simulink model "day04p2"  (R2026a)
settings: Solver=VariableStepAuto  StopTime=inf
undefined symbols (not defined in the file): DiscIntNeverNeededParam
libraries: simulink x6
(part 2 of 2)

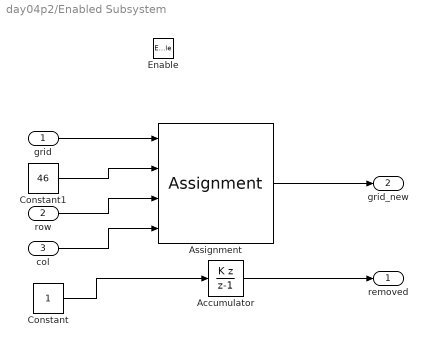
== system day04p2/Enabled Subsystem ==
  grid : Inport
  row : Inport  Port=2
  col : Inport  Port=3
  Enable : EnablePort
  Accumulator : DiscreteIntegrator  IntegratorMethod=Accumulation: Backward Euler  SampleTime=-1  ICPrevOutput=DiscIntNeverNeededParam  ICPrevScaledInput=DiscIntNeverNeededParam
  Assignment : Assignment  NumberOfDimensions=2  DiagnosticForDimensions=Warning  IndexOptions=Index vector (port),Index vector (port)  Indices=1,1  OutputSizes=1,1
  Constant : Constant
  Constant1 : Constant  Value=46
  removed : Outport
  grid_new : Outport  Port=2
  wires:
  Constant/1 -> Accumulator/1
  Accumulator/1 -> removed/1
  grid/1 -> Assignment/1
  Assignment/1 -> grid_new/1
  Constant1/1 -> Assignment/2
  row/1 -> Assignment/3
  col/1 -> Assignment/4

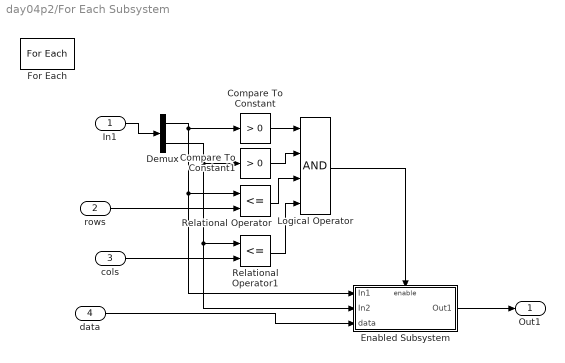
== system day04p2/For Each Subsystem ==
  In1 : Inport  Partition=on  PartitionDimension=1  PartitionWidth=1  PartitionOffset=0
  rows : Inport  Port=2
  cols : Inport  Port=3
  data : Inport  Port=4
  Compare To Constant : simulink/Logic and Bit Operations/Compare To Constant  relop=>  const=0  OutDataTypeStr=boolean
  Compare To Constant1 : simulink/Logic and Bit Operations/Compare To Constant  relop=>  const=0  OutDataTypeStr=boolean
  Demux : Demux  Outputs=2
  Enabled Subsystem : Subsystem  TreatAsAtomicUnit=on
  For Each : ForEach  DisableCoverage=on
  Logical Operator : Logic  Inputs=4  AllPortsSameDT=off  OutDataTypeStr=boolean
  Relational Operator : RelationalOperator  Operator=<=  OutDataTypeStr=boolean  RndMeth=Simplest  InputSameDT=off
  Relational Operator1 : RelationalOperator  Operator=<=  OutDataTypeStr=boolean  RndMeth=Simplest  InputSameDT=off
  Out1 : Outport  ConcatenationDimension=1
  wires:
  In1/1 -> Demux/1
  Demux/1 -> Enabled Subsystem/1(In1), Relational Operator/1, Compare To Constant/1
  Demux/2 -> Enabled Subsystem/2(In2), Relational Operator1/1, Compare To Constant1/1
  rows/1 -> Relational Operator/2
  cols/1 -> Relational Operator1/2
  Compare To Constant/1 -> Logical Operator/1
  Compare To Constant1/1 -> Logical Operator/2
  Relational Operator/1 -> Logical Operator/3
  Relational Operator1/1 -> Logical Operator/4
  data/1 -> Enabled Subsystem/3(data)
  Logical Operator/1 -> Enabled Subsystem/Enable
  Enabled Subsystem/1(Out1) -> Out1/1

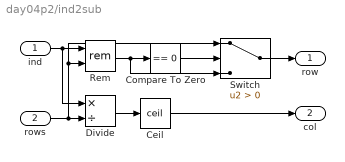
== system day04p2/ind2sub ==
  ind : Inport
  rows : Inport  Port=2
  Ceil : Rounding  Operator=ceil
  Compare To Zero : simulink/Logic and Bit Operations/Compare To Zero  relop===  OutDataTypeStr=boolean
  Divide : Product  Inputs=*/
  Rem : Math  Operator=rem
  Switch : Switch  Criteria=u2 > Threshold  SaturateOnIntegerOverflow=off  InputSameDT=off
  row : Outport
  col : Outport  Port=2
  wires:
  ind/1 -> Rem/1, Divide/1
  rows/1 -> Rem/2, Switch/1, Divide/2
  Divide/1 -> Ceil/1
  Ceil/1 -> col/1
  Rem/1 -> Switch/3, Compare To Zero/1
  Compare To Zero/1 -> Switch/2
  Switch/1 -> row/1

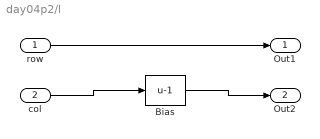
== system day04p2/l ==
  row : Inport
  col : Inport  Port=2
  Bias : Bias  Bias=-1  SaturateOnIntegerOverflow=off
  Out1 : Outport
  Out2 : Outport  Port=2
  wires:
  row/1 -> Out1/1
  col/1 -> Bias/1
  Bias/1 -> Out2/1

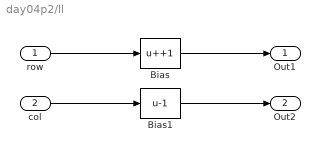
== system day04p2/ll ==
  row : Inport
  col : Inport  Port=2
  Bias : Bias  Bias=+1  SaturateOnIntegerOverflow=off
  Bias1 : Bias  Bias=-1  SaturateOnIntegerOverflow=off
  Out1 : Outport
  Out2 : Outport  Port=2
  wires:
  row/1 -> Bias/1
  Bias/1 -> Out1/1
  col/1 -> Bias1/1
  Bias1/1 -> Out2/1

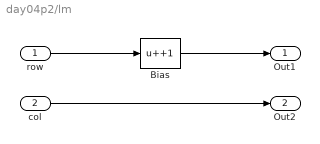
== system day04p2/lm ==
  row : Inport
  col : Inport  Port=2
  Bias : Bias  Bias=+1  SaturateOnIntegerOverflow=off
  Out1 : Outport
  Out2 : Outport  Port=2
  wires:
  row/1 -> Bias/1
  Bias/1 -> Out1/1
  col/1 -> Out2/1

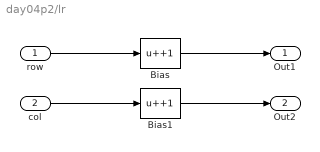
== system day04p2/lr ==
  row : Inport
  col : Inport  Port=2
  Bias : Bias  Bias=+1  SaturateOnIntegerOverflow=off
  Bias1 : Bias  Bias=+1  SaturateOnIntegerOverflow=off
  Out1 : Outport
  Out2 : Outport  Port=2
  wires:
  row/1 -> Bias/1
  Bias/1 -> Out1/1
  col/1 -> Bias1/1
  Bias1/1 -> Out2/1

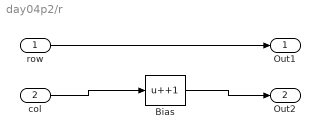
== system day04p2/r ==
  row : Inport
  col : Inport  Port=2
  Bias : Bias  Bias=+1  SaturateOnIntegerOverflow=off
  Out1 : Outport
  Out2 : Outport  Port=2
  wires:
  col/1 -> Bias/1
  Bias/1 -> Out2/1
  row/1 -> Out1/1

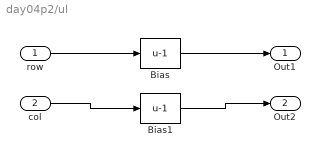
== system day04p2/ul ==
  row : Inport
  col : Inport  Port=2
  Bias : Bias  Bias=-1  SaturateOnIntegerOverflow=off
  Bias1 : Bias  Bias=-1  SaturateOnIntegerOverflow=off
  Out1 : Outport
  Out2 : Outport  Port=2
  wires:
  row/1 -> Bias/1
  Bias/1 -> Out1/1
  col/1 -> Bias1/1
  Bias1/1 -> Out2/1

== system day04p2/um ==
  row : Inport
  col : Inport  Port=2
  Bias : Bias  Bias=-1  SaturateOnIntegerOverflow=off
  Out1 : Outport
  Out2 : Outport  Port=2
  wires:
  col/1 -> Out2/1
  row/1 -> Bias/1
  Bias/1 -> Out1/1

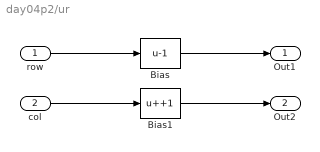
== system day04p2/ur ==
  row : Inport
  col : Inport  Port=2
  Bias : Bias  Bias=-1  SaturateOnIntegerOverflow=off
  Bias1 : Bias  Bias=+1  SaturateOnIntegerOverflow=off
  Out1 : Outport
  Out2 : Outport  Port=2
  wires:
  row/1 -> Bias/1
  Bias/1 -> Out1/1
  col/1 -> Bias1/1
  Bias1/1 -> Out2/1

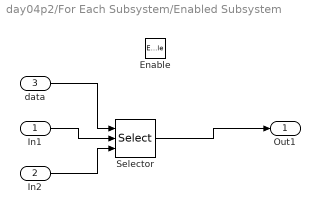
== system day04p2/For Each Subsystem/Enabled Subsystem ==
  In1 : Inport
  In2 : Inport  Port=2
  data : Inport  Port=3
  Enable : EnablePort
  Selector : Selector  NumberOfDimensions=2  InputPortWidth=3  IndexOptions=Index vector (port),Index vector (port)  Indices=[1 3],1  OutputSizes=1,1
  Out1 : Outport  OutputWhenDisabled=reset  InitialOutput=46
      settings: AttributesFormatString=|
      | %<OutputWhenDisabled>
      | %<InitialOutput>
  wires:
  In1/1 -> Selector/2
  In2/1 -> Selector/3
  Selector/1 -> Out1/1
  data/1 -> Selector/1
